simulink model "DormFridge"  (R2019a)
settings: Solver=VariableStepAuto  StartTime=0.0  StopTime=24.0  RelTol=1e-3
libraries: simulink x2
settings Model: OrderedModelArguments=off  Creator=champion  LastModifiedBy=champion

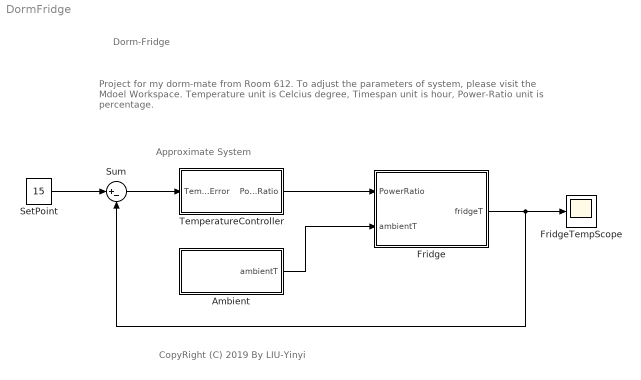
== system DormFridge ==
  note: Approximate System
  note: CopyRight (C) 2019 By LIU-Yinyi
  note: Project for my dorm-mate from Room 612.
      | To adjust the parameters of system, please visit the Mdoel Workspace.
      | Temperature unit is Celcius degree, Timespan unit is hour, Power-Ratio unit is percentage.
  note: Dorm-Fridge
  Ambient : Subsystem  mask(Simplified Ambient Environment Model){avgTemp=25, noiseRatio=10}
      mask prompts: avgTemp "AverageTemperature (C)"; noiseRatio "NoiseRatio (%)"
      mask help:
      | AverageTemperature unit is Celcius Degree.
      | NoiseRatio unit is percentage.
  Fridge : Subsystem  mask(Simplified Fridge Environment Model){coolerP=15, heatC=1004.5, equM=0.0008, kappa=0.691}
      mask prompts: coolerP "CoolerPower (W)"; heatC "HeatCapacity (J/kg·C)"; equM "EquivalentMass (kg)"; kappa "DissipationCoef (W/C)"
      mask help:
      | Use a simplified thermal model to simulate the fridge environment:
      | 1. CoolerPower is the maximum power of the Peltier Semiconductor.
      | 2. HeatCapacity is the simplified parameter of ideal model.
      | 3. EquivalentMass can be calculated by the product Gas Moore Volume and Gas Average Density.
      | 4. Kappa is an empirical constant.
      mask Help:
      | CoolerPower is the maximum power of the Peltier Semiconductor.
      | HeatCapacity and EquivalentMass are the simplified parameters of ideal model.
      | EquivalentMass can be calculated by the product Gas Moore Volume and Gas Average Density.
      | Kappa is an empirical constant.
  FridgeTempScope : Scope
  SetPoint : Constant  Value=15
  Sum : Sum  Inputs=|+-
  TemperatureController : Subsystem  mask(Temperature Controller){kP=8, kI=5, kD=0.7, kN=2}
      mask prompts: kP "Proportion"; kI "Integral"; kD "Deviation"; kN "FilterCoef"
      mask help: Simple parallel PID controller with respect to temperature.
      mask Help: Enter PID coefficients in the block diagram.
  wires:
  SetPoint/1 -> Sum/1
  Sum/1 -> TemperatureController/1(TempError)
  Ambient/1(ambientT) -> Fridge/2(ambientT)
  TemperatureController/1(PowerRatio) -> Fridge/1(PowerRatio)
  Fridge/1(fridgeT) -> FridgeTempScope/1, Sum/2

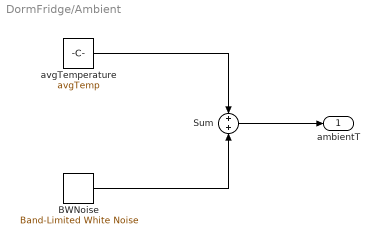
== system DormFridge/Ambient ==
  BWNoise : simulink/Sources/Band-Limited White Noise  Cov=[noiseRatio/100]  Ts=0.1  seed=[23341]
  Sum : Sum
  avgTemperature : Constant  Value=avgTemp
  ambientT : Outport
  wires:
  Sum/1 -> ambientT/1
  avgTemperature/1 -> Sum/1
  BWNoise/1 -> Sum/2

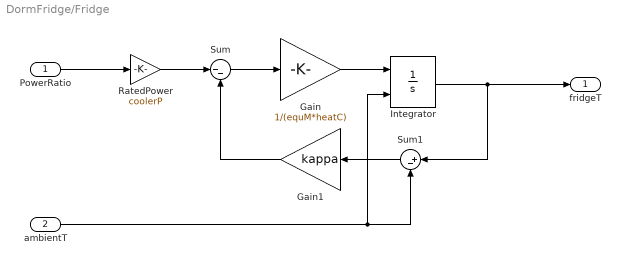
== system DormFridge/Fridge ==
  PowerRatio : Inport
  ambientT : Inport  Port=2
  Gain : Gain  Gain=1/(equM*heatC)
  Gain1 : Gain  Gain=kappa
  Integrator : Integrator  InitialConditionSource=external
  RatedPower : Gain  Gain=coolerP
  Sum : Sum  Inputs=|--
  Sum1 : Sum  Inputs=|+-
  fridgeT : Outport
  wires:
  Sum/1 -> Gain/1
  Gain/1 -> Integrator/1
  Integrator/1 -> Sum1/1, fridgeT/1
  Sum1/1 -> Gain1/1
  ambientT/1 -> Sum1/2, Integrator/2
  Gain1/1 -> Sum/2
  PowerRatio/1 -> RatedPower/1
  RatedPower/1 -> Sum/1

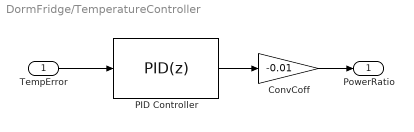
== system DormFridge/TemperatureController ==
  TempError : Inport
  ConvCoff : Gain  Gain=-0.01
  PID Controller : simulink/Continuous/PID Controller  Controller=PID  Form=Parallel  TimeDomain=Discrete-time  SampleTime=-1  IntegratorMethod=Forward Euler  FilterMethod=Forward Euler  ControllerParametersSource=internal  P=kP  I=kI  D=kD  UseFilter=on  N=kN  TunerSelectOption=Transfer Function Based (PID Tuner App)  InitialConditionSource=internal  InitialConditionForIntegrator=0  InitialConditionForFilter=0  DifferentiatorICPrevScaledInput=0  ExternalReset=none  TrackingMode=off  Kt=1  LimitOutput=on  UpperSaturationLimit=0  LowerSaturationLimit=-100  LinearizeAsGain=on  AntiWindupMode=none  Kb=1  POutMin=[]  POutMax=[]  IOutMin=[]  IOutMax=[]  DOutMin=[]  DOutMax=[]  NOutMin=[]  NOutMax=[]  SumOutMin=[]  SumOutMax=[]  SaturationOutMin=[]  SaturationOutMax=[]  PParamMin=[]  PParamMax=[]  IParamMin=[]  IParamMax=[]  DParamMin=[]  DParamMax=[]  NParamMin=[]  NParamMax=[]  KbParamMin=[]  KbParamMax=[]  KtParamMin=[]  KtParamMax=[]  KbOutMin=[]  KbOutMax=[]  KtOutMin=[]  KtOutMax=[]  IntegratorOutMin=[]  IntegratorOutMax=[]  FilterOutMin=[]  FilterOutMax=[]  SumI1OutMin=[]  SumI1OutMax=[]  SumI2OutMin=[]  SumI2OutMax=[]  SumI3OutMin=[]  SumI3OutMax=[]  SumI4OutMin=[]  SumI4OutMax=[]  SumDOutMin=[]  SumDOutMax=[]  DifferentiatorOutMin=[]  DifferentiatorOutMax=[]  FilterDiffOutCoefMin=[]  FilterDiffOutCoefMax=[]  ReciprocalOutMin=[]  ReciprocalOutMax=[]  SumDenOutMin=[]  SumDenOutMax=[]  SumNumOutMin=[]  SumNumOutMax=[]  DivideOutMin=[]  DivideOutMax=[]  IntegratorContinuousStateAttributes=''  IntegratorStateMustResolveToSignalObject=off  IntegratorRTWStateStorageClass=Auto  FilterContinuousStateAttributes=''  FilterStateMustResolveToSignalObject=off  FilterRTWStateStorageClass=Auto  ParallelPVariant=InternalParameters  IdealPVariant=Disabled  IVariant=InternalParameters  DVariant=InternalParameters  IntegratorVariant=Discrete  SatVariant=Enabled  AWVariant=Passthrough  PCopyVariant=Disabled  TRVariant=Disabled  FdbkBlocksVariant=Forward  IdealPFdbkVariant=Disabled  SatFdbkVariant=Disabled  DerivativeFilterVariant=ForwardEulerFilter  NVariant=InternalParameters  NCopyVariant=Disabled  FilterICVariant=InternalICsFilter  IntegratorICVariant=InternalICs  ExternalResetVariant=Disabled  TRSumVariant=Passthrough  SumFdbkVariant=Disabled  SumVariant=Sum_PID
  PowerRatio : Outport
  wires:
  TempError/1 -> PID Controller/1
  PID Controller/1 -> ConvCoff/1
  ConvCoff/1 -> PowerRatio/1
